simulink model "dynamics"  (R2021b)
settings: Solver=ode15s  StartTime=0.0  StopTime=6.1  RelTol=1e-5
undefined symbols (not defined in the file or in its folder): f_fcn
settings Model: Creator=cosimodellasantina  LastModifiedBy=mrsub
settings SolverCC: AlgebraicLoopSolver=TrustRegion
settings DebuggingCC: SFMachineParentedDataDiag=warning
settings SFSimCC: CustomCodeUndefinedFunction=UseInterfaceOnly

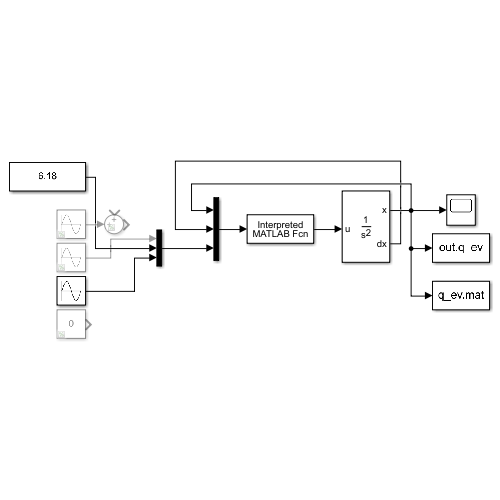
[thumbnail: Simulink's stored preview of the top-level diagram]
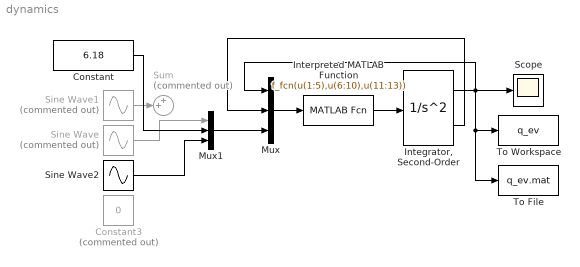
== system dynamics ==
  Constant : Constant  Value=6.18
  Constant3 : Constant  Commented=on  Value=0
  "Integrator, Second-Order" : SecondOrderIntegrator  ICX=x_0  ICDXDT=dx_0
  Interpreted MATLAB Function : MATLABFcn  MATLABFcn=f_fcn(u(1:5),u(6:10),u(11:13))
  Mux : Mux  Inputs=3
  Mux1 : Mux  Inputs=3
  Scope : Scope
  Sine Wave : Sin  Commented=on  Frequency=pi  SampleTime=0
  Sine Wave1 : Sin  Commented=on  Amplitude=0  Frequency=pi  SampleTime=0
  Sine Wave2 : Sin  Amplitude=0.2  Frequency=2*pi  SampleTime=0
  Sum : Sum  Commented=on  Inputs=++|
  To File : ToFile  Filename=q_ev.mat  SaveFormat=Timeseries
  To Workspace : ToWorkspace  VariableName=q_ev  SaveFormat=Timeseries  SampleTime=-1
  wires:
  Mux/1 -> Interpreted MATLAB Function/1
  Interpreted MATLAB Function/1 -> "Integrator, Second-Order"/1
  "Integrator, Second-Order"/1 -> Mux/1, To File/1, To Workspace/1, Scope/1
  Sine Wave1/1 -> Sum/2
  Mux1/1 -> Mux/3
  "Integrator, Second-Order"/2 -> Mux/2
  Sine Wave/1 -> Mux1/1
  Constant/1 -> Mux1/2
  Sine Wave2/1 -> Mux1/3
